simulink model "DOF6_Trajectory_simulation"  (R2018b)
settings: Solver=FixedStepAuto  StartTime=0.0  StopTime=60  FixedStep=0.05  RelTol=1e-3
undefined symbols (not defined in the file or in its folder): ace_var, pos_var, spe_var
settings Model: Creator=root  LastModifiedBy=root

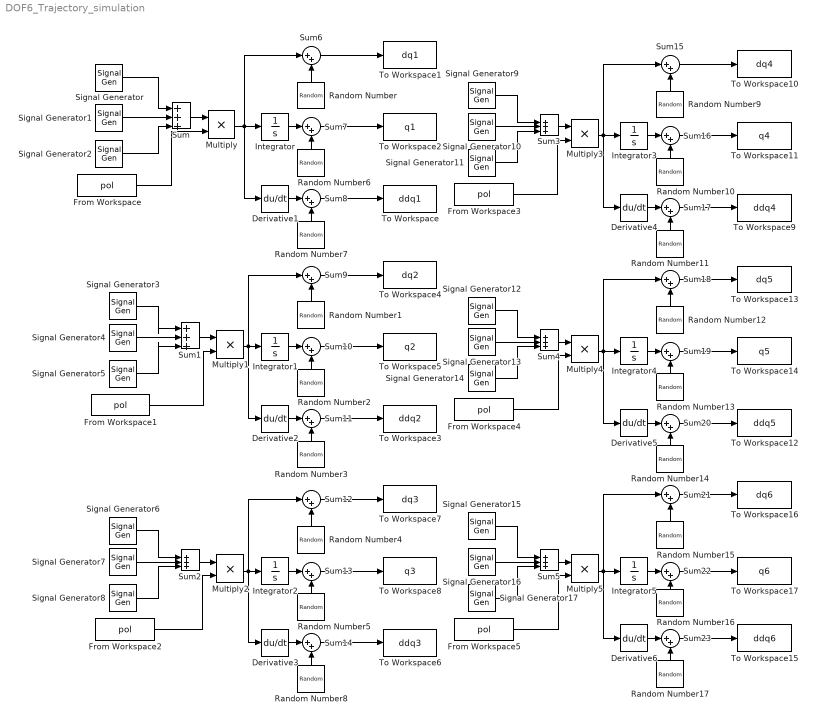
== system DOF6_Trajectory_simulation ==
  Derivative{1..6} (6 alike) : Derivative
  From Workspace{,3..5} (4 alike) : FromWorkspace  VariableName=pol
  From Workspace1 : FromWorkspace  VariableName=pol  SampleTime=0
  From Workspace2 : FromWorkspace  VariableName=pol  SampleTime=0
  Integrator{,1..5} (6 alike) : Integrator
  Multiply{,1..5} (6 alike) : Product
  Random Number : RandomNumber  Variance=spe_var
  Random Number1 : RandomNumber  Variance=spe_var  Seed=3
  Random Number10 : RandomNumber  Variance=pos_var  Seed=10
  Random Number11 : RandomNumber  Variance=ace_var  Seed=11
  Random Number12 : RandomNumber  Variance=spe_var  Seed=12
  Random Number13 : RandomNumber  Variance=pos_var  Seed=13
  Random Number14 : RandomNumber  Variance=ace_var  Seed=14
  Random Number15 : RandomNumber  Variance=spe_var  Seed=15
  Random Number16 : RandomNumber  Variance=pos_var  Seed=16
  Random Number17 : RandomNumber  Variance=ace_var  Seed=17
  Random Number2 : RandomNumber  Variance=pos_var  Seed=4
  Random Number3 : RandomNumber  Variance=ace_var  Seed=5
  Random Number4 : RandomNumber  Variance=spe_var  Seed=6
  Random Number5 : RandomNumber  Variance=pos_var  Seed=7
  Random Number6 : RandomNumber  Variance=pos_var  Seed=1
  Random Number7 : RandomNumber  Variance=ace_var  Seed=2
  Random Number8 : RandomNumber  Variance=ace_var  Seed=8
  Random Number9 : RandomNumber  Variance=spe_var  Seed=9
  Signal Generator : SignalGenerator  Amplitude=0.12  Frequency=1.25  Units=rad/sec
  Signal Generator1 : SignalGenerator  Amplitude=0.12  Frequency=0.95  Units=rad/sec
  Signal Generator10 : SignalGenerator  Amplitude=-0.1  Units=rad/sec
  Signal Generator11 : SignalGenerator  Amplitude=-0.1  Frequency=0.4  Units=rad/sec
  Signal Generator12 : SignalGenerator  Amplitude=0.12  Units=rad/sec
  Signal Generator13 : SignalGenerator  Amplitude=0.12  Frequency=0.66  Units=rad/sec
  Signal Generator14 : SignalGenerator  Amplitude=0.12  Frequency=0.33  Units=rad/sec
  Signal Generator15 : SignalGenerator  Amplitude=0.3  Frequency=0.45  Units=rad/sec
  Signal Generator16 : SignalGenerator  Amplitude=0.3  Frequency=0.5  Units=rad/sec
  Signal Generator17 : SignalGenerator  Amplitude=0.3  Frequency=0.125  Units=rad/sec
  Signal Generator2 : SignalGenerator  Amplitude=-0.15  Units=rad/sec
  Signal Generator3 : SignalGenerator  Amplitude=0.1  Frequency=1.3  Units=rad/sec
  Signal Generator4 : SignalGenerator  Amplitude=0.1  Frequency=0.85  Units=rad/sec
  Signal Generator5 : SignalGenerator  Amplitude=-0.12  Frequency=0.25  Units=rad/sec
  Signal Generator6 : SignalGenerator  Amplitude=0.1  Frequency=2.5  Units=rad/sec
  Signal Generator7 : SignalGenerator  Amplitude=0.1  Frequency=2  Units=rad/sec
  Signal Generator8 : SignalGenerator  Amplitude=0.1  Frequency=0.85  Units=rad/sec
  Signal Generator9 : SignalGenerator  Amplitude=0.2  Frequency=0.4  Units=rad/sec
  Sum{,1..5} (6 alike) : Sum  Inputs=|+++
  Sum{6..23} (18 alike) : Sum  Inputs=|++
  To Workspace : ToWorkspace  VariableName=ddq1  SampleTime=-1
  To Workspace1 : ToWorkspace  VariableName=dq1  SampleTime=-1
  To Workspace10 : ToWorkspace  VariableName=dq4  SampleTime=-1
  To Workspace11 : ToWorkspace  VariableName=q4  SampleTime=-1
  To Workspace12 : ToWorkspace  VariableName=ddq5  SampleTime=-1
  To Workspace13 : ToWorkspace  VariableName=dq5  SampleTime=-1
  To Workspace14 : ToWorkspace  VariableName=q5  SampleTime=-1
  To Workspace15 : ToWorkspace  VariableName=ddq6  SampleTime=-1
  To Workspace16 : ToWorkspace  VariableName=dq6  SampleTime=-1
  To Workspace17 : ToWorkspace  VariableName=q6  SampleTime=-1
  To Workspace2 : ToWorkspace  VariableName=q1  SampleTime=-1
  To Workspace3 : ToWorkspace  VariableName=ddq2  SampleTime=-1
  To Workspace4 : ToWorkspace  VariableName=dq2  SampleTime=-1
  To Workspace5 : ToWorkspace  VariableName=q2  SampleTime=-1
  To Workspace6 : ToWorkspace  VariableName=ddq3  SampleTime=-1
  To Workspace7 : ToWorkspace  VariableName=dq3  SampleTime=-1
  To Workspace8 : ToWorkspace  VariableName=q3  SampleTime=-1
  To Workspace9 : ToWorkspace  VariableName=ddq4  SampleTime=-1
  wires:
  Signal Generator/1 -> Sum/1
  Signal Generator1/1 -> Sum/2
  Signal Generator2/1 -> Sum/3
  Signal Generator5/1 -> Sum1/3
  Signal Generator3/1 -> Sum1/1
  Signal Generator4/1 -> Sum1/2
  Signal Generator8/1 -> Sum2/3
  Signal Generator6/1 -> Sum2/1
  Signal Generator7/1 -> Sum2/2
  Signal Generator11/1 -> Sum3/3
  Signal Generator9/1 -> Sum3/1
  Signal Generator10/1 -> Sum3/2
  Signal Generator14/1 -> Sum4/3
  Signal Generator12/1 -> Sum4/1
  Signal Generator13/1 -> Sum4/2
  Signal Generator17/1 -> Sum5/3
  Signal Generator15/1 -> Sum5/1
  Signal Generator16/1 -> Sum5/2
  From Workspace/1 -> Multiply/2
  Sum/1 -> Multiply/1
  From Workspace1/1 -> Multiply1/2
  Sum1/1 -> Multiply1/1
  Sum2/1 -> Multiply2/1
  From Workspace2/1 -> Multiply2/2
  Sum3/1 -> Multiply3/1
  From Workspace3/1 -> Multiply3/2
  Sum4/1 -> Multiply4/1
  From Workspace4/1 -> Multiply4/2
  Sum5/1 -> Multiply5/1
  From Workspace5/1 -> Multiply5/2
  Multiply/1 -> Derivative1/1, Sum6/1, Integrator/1
  Sum6/1 -> To Workspace1/1
  Integrator/1 -> Sum7/1
  Random Number6/1 -> Sum7/2
  Sum7/1 -> To Workspace2/1
  Random Number/1 -> Sum6/2
  Random Number7/1 -> Sum8/2
  Derivative1/1 -> Sum8/1
  Sum8/1 -> To Workspace/1
  Integrator1/1 -> Sum10/1
  Random Number3/1 -> Sum11/2
  Multiply1/1 -> Derivative2/1, Sum9/1, Integrator1/1
  Random Number2/1 -> Sum10/2
  Derivative2/1 -> Sum11/1
  Random Number1/1 -> Sum9/2
  Sum11/1 -> To Workspace3/1
  Sum10/1 -> To Workspace5/1
  Sum9/1 -> To Workspace4/1
  Integrator2/1 -> Sum13/1
  Random Number8/1 -> Sum14/2
  Multiply2/1 -> Derivative3/1, Integrator2/1, Sum12/1
  Random Number5/1 -> Sum13/2
  Derivative3/1 -> Sum14/1
  Random Number4/1 -> Sum12/2
  Sum14/1 -> To Workspace6/1
  Sum13/1 -> To Workspace8/1
  Sum12/1 -> To Workspace7/1
  Multiply3/1 -> Integrator3/1, Derivative4/1, Sum15/1
  Integrator3/1 -> Sum16/1
  Random Number11/1 -> Sum17/2
  Random Number10/1 -> Sum16/2
  Derivative4/1 -> Sum17/1
  Random Number9/1 -> Sum15/2
  Sum17/1 -> To Workspace9/1
  Sum16/1 -> To Workspace11/1
  Sum15/1 -> To Workspace10/1
  Integrator4/1 -> Sum19/1
  Random Number14/1 -> Sum20/2
  Multiply4/1 -> Derivative5/1, Sum18/1, Integrator4/1
  Random Number13/1 -> Sum19/2
  Derivative5/1 -> Sum20/1
  Random Number12/1 -> Sum18/2
  Sum20/1 -> To Workspace12/1
  Sum19/1 -> To Workspace14/1
  Sum18/1 -> To Workspace13/1
  Multiply5/1 -> Integrator5/1, Sum21/1, Derivative6/1
  Integrator5/1 -> Sum22/1
  Random Number17/1 -> Sum23/2
  Random Number16/1 -> Sum22/2
  Derivative6/1 -> Sum23/1
  Random Number15/1 -> Sum21/2
  Sum22/1 -> To Workspace17/1
  Sum21/1 -> To Workspace16/1
  Sum23/1 -> To Workspace15/1
